simulink model "DC_Motor_Control_with_3_Phase_Converter"  (R2021b)
settings: Solver=ode23t  StartTime=0.0  StopTime=4  MaxStep=0.0055632823365785811  RelTol=1e-3
undefined symbols (not defined in the file): D1, lagging, pulse
libraries: spsACVoltageSourceLib x3, spsSeriesRLCBranchLib x2, spsCurrentMeasurementLib x1, spsDCMachineLib x1, spsDCVoltageSourceLib x1, spsGroundLib x1, spsPLL3phLib x1, spsPulseGeneratorThyristor6PulseLib x1, spsThreePhaseVIMeasurementLib x1, spsUniversalBridgeLib x1, spsVoltageMeasurementLib x1, spspowerguiLib x1
settings Model: Creator=piyus  LastModifiedBy=psvac
settings SolverCC: ZeroCrossAlgorithm=Adaptive
settings DebuggingCC: IgnoredZcDiagnostic=none  UnconnectedInputMsg=none  UnconnectedOutputMsg=none  UnconnectedLineMsg=none
settings ModelReferenceCC: EnableRefExpFcnMdlSchedulingChecks=off
settings RTWCC: DLArmComputeVersion=20.02.1

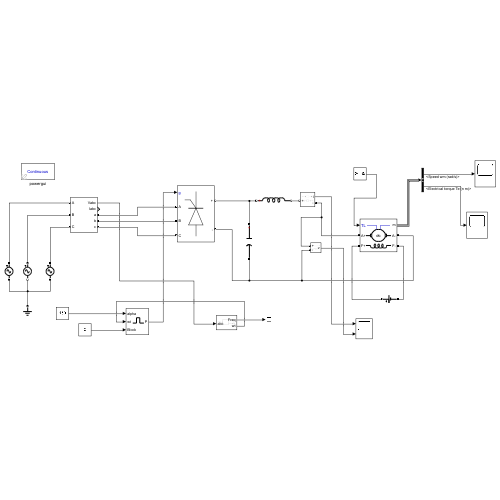
[thumbnail: Simulink's stored preview of the top-level diagram]
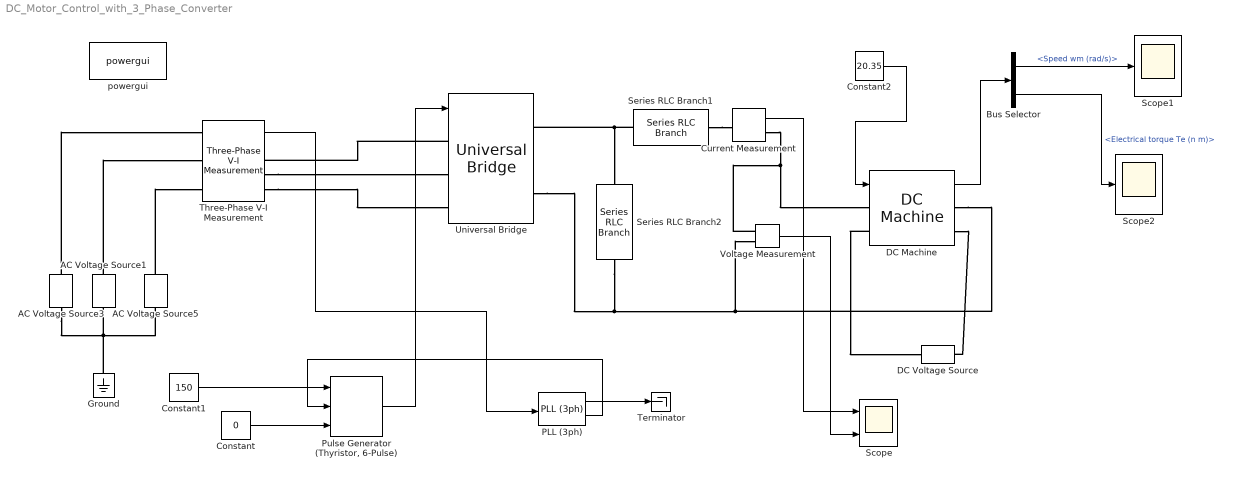
== system DC_Motor_Control_with_3_Phase_Converter ==
  AC Voltage Source1 : spsACVoltageSourceLib/AC Voltage Source  Amplitude=141  Phase=120  Frequency=60  SampleTime=0  Measurements=None  BusType=swing  Pref=10e3  Qref=0  Qmin=-inf  Qmax=+inf
  AC Voltage Source3 : spsACVoltageSourceLib/AC Voltage Source  Amplitude=141  Phase=0  Frequency=60  SampleTime=0  Measurements=None  BusType=swing  Pref=10e3  Qref=0  Qmin=-inf  Qmax=+inf
  AC Voltage Source5 : spsACVoltageSourceLib/AC Voltage Source  Amplitude=141  Phase=240  Frequency=60  SampleTime=0  Measurements=None  BusType=swing  Pref=10e3  Qref=0  Qmin=-inf  Qmax=+inf
  Bus Selector : BusSelector  OutputSignals=Speed wm (rad/s),Electrical torque Te (n m)
  Constant : Constant  Value=0
  Constant1 : Constant  Value=150
  Constant2 : Constant  Value=20.35
  Current Measurement : spsCurrentMeasurementLib/Current Measurement  PhasorSimulation=off  OutputType=Complex  PSBequivalent=0
  DC Machine : spsDCMachineLib/DC Machine  PresetModel=01: 5HP 240V 1750RPM Field:300V  MechanicalLoad=Torque TL  FieldType=Wound  ShowDetailedParameters=on  MeasurementBus=off  RLa=[2.581 0.028]  RLf=[281.2 156]  Laf=0.9483  MachineConstant=Torque constant (N.m/A)  Ke=1.8  Kt=1.8  J=0.02215  Bm=0.002953  Tf=0.5161  w0=1  Ifinit=1.06685633001422  TsPowergui=0  TsBlock=-1
  DC Voltage Source : spsDCVoltageSourceLib/DC Voltage Source  Amplitude=300  Measurements=None
  Ground : spsGroundLib/Ground  LConnTagsString=a
  PLL (3ph) : spsPLL3phLib/PLL (3ph)  Fmin=45  Par_Init=[0, 60]  ParK=[180, 3200, 1]  TcD=1e-4  MaxRateChangeFreq=12  FilterCutOffFreq=25  Ts=0  AGC=on
  "Pulse Generator (Thyristor, 6-Pulse)" : spsPulseGeneratorThyristor6PulseLib/Pulse Generator (Thyristor, 6-Pulse)  GenType=6-pulse  Delta=D1 (lagging)  pwidth=60  Double_Pulse=off  Ts=0
      settings: SourceProductBaseCode=PS
  Scope : Scope  NumInputPorts=2
  Scope1 : Scope
  Scope2 : Scope
  Series RLC Branch1 : spsSeriesRLCBranchLib/Series RLC Branch  LConnTagsString=__new0  RConnTagsString=__new0  BranchType=L  Resistance=0  Inductance=500e-3  SetiL0=off  InitialCurrent=0  Capacitance=0  Setx0=off  InitialVoltage=0  Measurements=None
  Series RLC Branch2 : spsSeriesRLCBranchLib/Series RLC Branch  LConnTagsString=__new0  RConnTagsString=__new0  BranchType=C  Resistance=0  Inductance=0  SetiL0=off  InitialCurrent=0  Capacitance=7000e-6  Setx0=off  InitialVoltage=0  Measurements=None
  Terminator : Terminator
  Three-Phase V-I Measurement : spsThreePhaseVIMeasurementLib/Three-Phase V-I Measurement  VoltageMeasurement=phase-to-ground  SetLabelV=off  LabelV=Vabc  Vpu=off  VpuLL=off  CurrentMeasurement=yes  SetLabelI=off  LabelI=Iabc  Ipu=off  Pbase=100e6  Vbase=500e3  OutputType=Complex  PhasorSimulation=off  PSBequivalent=0
  Universal Bridge : spsUniversalBridgeLib/Universal Bridge  Arms=3  SnubberResistance=1e5  SnubberCapacitance=inf  Device=Thyristors  Ron=1e-3  Lon=0  ForwardVoltages="[  0  0  ]"  ForwardVoltage=0  GTOparameters=[ 10e-6 , 20e-6 ]  IGBTparameters=[ 1e-6 , 2e-6 ]  Measurements=None  Measurements_2=None  converterType=Rectifier
  Voltage Measurement : spsVoltageMeasurementLib/Voltage Measurement  PhasorSimulation=off  OutputType=Complex  PSBequivalent=0
  powergui : spspowerguiLib/powergui  Priority=1  SimulationMode=Continuous  SampleTime=50e-6  frequency=60  Iterations=50  frequencyindice=60  Pbase=100e6  ErrMax=1e-4  UnitsV=kV  UnitsW=MW  buscounter=0  FunctionMessages=off  echomessages=off  EnableUseOfTLC=off  CurrentSourceSwitches=off  DisableSnubberDevices=off  DisableRonSwitches=off  DisableVfSwitches=off  DisplayEquations=off  AutomaticDiscreteSolvers=off  SolverType=Tustin/Backward Euler (TBE)  Interpol=off  ExternalGateDelay=off  methode=off  Ts=100  x0status=blocks  SPID=on  SwTol=0  HookPort=off  NonlinearTolerance=1e-4  nMaxIteration=100  ContinueOnMaxIteration=off  RestoreLinks=warning  ResistiveCurrentMeasurement=off  Frange=[0:2:500]  Ylog=off  Xlog=on  ShowGrid=off  save=off  variable=ZData  structure=0  ZoomFFT=off  StartTime=0.0  cycles=1  DisplayStyle=1  fundamental=60  FreqAxis=off  MaxFrequency=1000  frequencyindicesteady=1  RmsSteady=1  display=off
  wires:
  Constant/1 -> "Pulse Generator (Thyristor, 6-Pulse)"/3
  Constant1/1 -> "Pulse Generator (Thyristor, 6-Pulse)"/1
  Three-Phase V-I Measurement/1 -> PLL (3ph)/1
  PLL (3ph)/1 -> Terminator/1
  PLL (3ph)/2 -> "Pulse Generator (Thyristor, 6-Pulse)"/2
  Voltage Measurement/1 -> Scope/2
  Current Measurement/1 -> Scope/1
  "Pulse Generator (Thyristor, 6-Pulse)"/1 -> Universal Bridge/1
  Constant2/1 -> DC Machine/1
  DC Machine/1 -> Bus Selector/1
  Bus Selector/1 -> Scope1/1  "<Speed wm (rad/s)>"
  Bus Selector/2 -> Scope2/1  "<Electrical torque Te (n m)>"
  connections:
  AC Voltage Source3/LConn1 -- AC Voltage Source5/LConn1 -- Ground/LConn1 -- AC Voltage Source1/LConn1
  AC Voltage Source3/RConn1 -- Three-Phase V-I Measurement/LConn1
  AC Voltage Source1/RConn1 -- Three-Phase V-I Measurement/LConn2
  AC Voltage Source5/RConn1 -- Three-Phase V-I Measurement/LConn3
  Universal Bridge/LConn1 -- Three-Phase V-I Measurement/RConn1
  Three-Phase V-I Measurement/RConn2 -- Universal Bridge/LConn2
  Three-Phase V-I Measurement/RConn3 -- Universal Bridge/LConn3
  Current Measurement/RConn1 -- Voltage Measurement/LConn1 -- DC Machine/LConn1
  Universal Bridge/RConn2 -- DC Machine/RConn1 -- Voltage Measurement/LConn2 -- Series RLC Branch2/RConn1
  Series RLC Branch1/LConn1 -- Universal Bridge/RConn1 -- Series RLC Branch2/LConn1
  Series RLC Branch1/RConn1 -- Current Measurement/LConn1
  DC Machine/LConn2 -- DC Voltage Source/RConn1
  DC Machine/RConn2 -- DC Voltage Source/LConn1
